simulink model "MSAS Project Part 2.2"  (R2023b)
settings: Solver=ode15s  StartTime=0.0  StopTime=Period  RelTol=1e-9  AbsTol=1e-9
undefined symbols (not defined in the file or in its folder): accelerometer, amplifier, drag, thruster, valve
libraries: fl_lib x15, nesl_utility x10, ee_lib x1
settings Model: Creator=matte  LastModifiedBy=matte

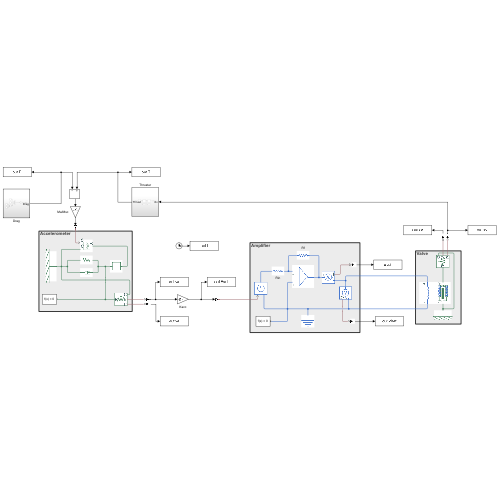
[thumbnail: Simulink's stored preview of the top-level diagram]
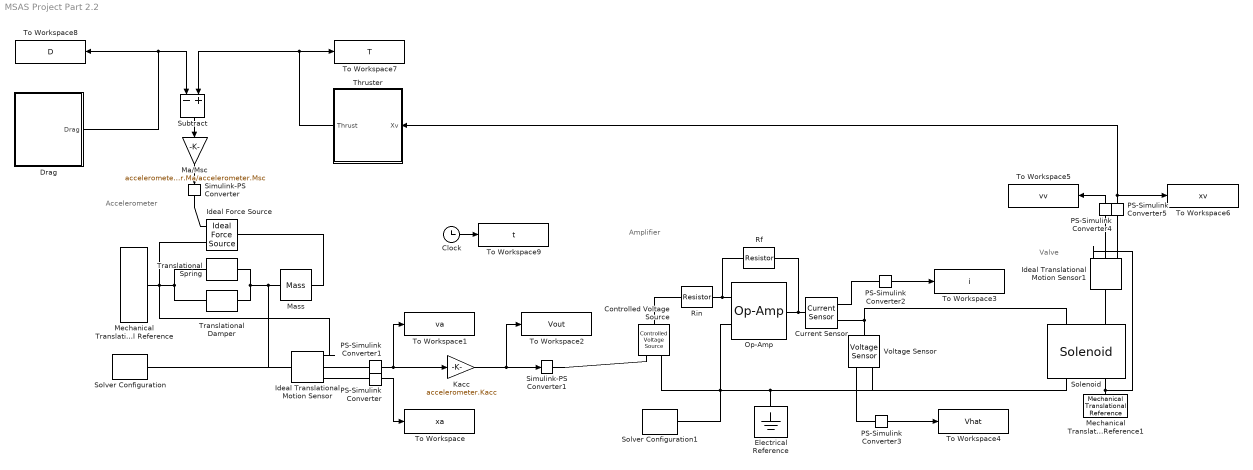
== system MSAS Project Part 2.2 ==
  note: Valve
  note: Amplifier
  note: Accelerometer
  Clock : Clock
  Controlled Voltage Source : fl_lib/Electrical/Electrical Sources/Controlled Voltage Source
  Current Sensor : fl_lib/Electrical/Electrical Sensors/Current Sensor
  Drag : Subsystem
  Electrical Reference : fl_lib/Electrical/Electrical Elements/Electrical Reference
  Ideal Force Source : fl_lib/Mechanical/Mechanical Sources/Ideal Force Source
  Ideal Translational Motion Sensor : fl_lib/Mechanical/Mechanical Sensors/Ideal Translational Motion Sensor  reference=foundation.enum.MeasurementReference.difference  acceleration_port=false  velocity_port=true  position_port=true  offset=0 m
  Ideal Translational Motion Sensor1 : fl_lib/Mechanical/Mechanical Sensors/Ideal Translational Motion Sensor  reference=foundation.enum.MeasurementReference.difference  acceleration_port=false  velocity_port=true  position_port=true  offset=0 m
  Kacc : Gain  Gain=accelerometer.Kacc
  Ma/Msc : Gain  Gain=accelerometer.Ma/accelerometer.Msc
  Mass : fl_lib/Mechanical/Translational Elements/Mass  mass=accelerometer.Ma kg  num_ports=foundation.enum.numPorts2.two  v_specify=off  v_priority=High  v=0 m/s  v_nominal_specify=off  v_nominal_unit=m/s  v_nominal_value=1  f_specify=off  f_priority=None  f=0 N  f_nominal_specify=off  f_nominal_unit=N  f_nominal_value=1
      settings: InternalSimscapePortConfiguration="{\"Bottom\":[],\"Left\":[{\"id\":\"M\",\"label\":\"\",\"type\":\"foundation.mechanical.translational.translational\"}],\"Right\":[{\"id\":\"N\",\"label\":\"\",\"type\":\"foundation.mechanical.translational.translational\"}],\"Top\":[]}"
  Mechanical Translational Reference : fl_lib/Mechanical/Translational Elements/Mechanical Translational Reference
  Mechanical Translational Reference1 : fl_lib/Mechanical/Translational Elements/Mechanical Translational Reference
  Op-Amp : fl_lib/Electrical/Electrical Elements/Op-Amp  outI_specify=off  outI_priority=None  outI=0 A  outI_nominal_specify=off  outI_nominal_unit=A  outI_nominal_value=1
  PS-Simulink Converter{,1..5} (6 alike) : nesl_utility/PS-Simulink Converter  PhysicalDomain=network_engine_domain  SubClassName=ps_output  LeftPortType=input  RightPortType=output  PseudoPeriodic=off  Frequencies=[]  VectorFormat=inherit  Unit=inherit  AffineConversion=off
  Rf : fl_lib/Electrical/Electrical Elements/Resistor  R=amplifier.Rf Ohm  i_specify=off  i_priority=None  i=0 A  i_nominal_specify=off  i_nominal_unit=A  i_nominal_value=1  v_specify=off  v_priority=None  v=0 V  v_nominal_specify=off  v_nominal_unit=V  v_nominal_value=1
  Rin : fl_lib/Electrical/Electrical Elements/Resistor  R=amplifier.Rin Ohm  i_specify=off  i_priority=None  i=0 A  i_nominal_specify=off  i_nominal_unit=A  i_nominal_value=1  v_specify=off  v_priority=None  v=0 V  v_nominal_specify=off  v_nominal_unit=V  v_nominal_value=1
  Simulink-PS Converter : nesl_utility/Simulink-PS Converter  PhysicalDomain=network_engine_domain  SubClassName=ps_input  LeftPortType=input  RightPortType=output  PseudoPeriodic=off  Frequencies=[]  NoiseDistribution=none  NoiseParameters=[]  Unit=1  AffineConversion=off  FilteringAndDerivatives=provide  SimscapeFilterOrder=1  InputFilterTimeConstant=0.001  UdotUserProvided=0
  Simulink-PS Converter1 : nesl_utility/Simulink-PS Converter  PhysicalDomain=network_engine_domain  SubClassName=ps_input  LeftPortType=input  RightPortType=output  PseudoPeriodic=off  Frequencies=[]  NoiseDistribution=none  NoiseParameters=[]  Unit=1  AffineConversion=off  FilteringAndDerivatives=provide  SimscapeFilterOrder=1  InputFilterTimeConstant=0.001  UdotUserProvided=0
  Solenoid : ee_lib/Electromechanical/Mechatronic Actuators/Solenoid  motionDirection=ee.enum.actuators.solenoidDirection.away  F12=[9000, 12] N  X12=[0, 0.1] mm  Vdc=0.6 mV  Imax=0.1 A  K=valve.kv N/m  Xzero=valve.xvMax m  lam=valve.bv N*s/m  Mass=valve.Mv kg  Xmax=0.1 mm  K_endstop=0.12*1e6 N/m  D_endstop=1e4 N*s/m  i_specify=on  i_priority=High  i=0 A  i_nominal_specify=off  i_nominal_unit=A  i_nominal_value=1  x_specify=on  x_priority=High  x=valve.xvMax m  x_nominal_specify=on  x_nominal_unit=m  x_nominal_value=valve.xvMax  vel_specify=off  vel_priority=None  vel=0 mm/s  vel_nominal_specify=off  vel_nominal_unit=mm/s  vel_nominal_value=1  F_specify=off  F_priority=None  F=0 N  F_nominal_specify=off  F_nominal_unit=N  F_nominal_value=1  v_L_specify=off  v_L_priority=None  v_L=0 V  v_L_nominal_specify=off  v_L_nominal_unit=V  v_L_nominal_value=1  magnetic_force_specify=off  magnetic_force_priority=None  magnetic_force=0 N  magnetic_force_nominal_specify=off  magnetic_force_nominal_unit=N  magnetic_force_nominal_value=1  alpha=3.93e-3 1/K  Tmeas=25 degC  thermal_mass=100 J/K  temperature_specify=off  temperature_priority=High  temperature=25 degC  temperature_nominal_specify=off  temperature_nominal_unit=degC  temperature_nominal_value=1  Q_specify=off  Q_priority=None  Q=0 W  Q_nominal_specify=off  Q_nominal_unit=W  Q_nominal_value=1
      settings: InternalSimscapePortConfiguration="{\"Bottom\":[],\"Left\":[{\"id\":\"p\",\"label\":\"+\",\"type\":\"foundation.electrical.electrical\"},{\"id\":\"R\",\"label\":\"R\",\"type\":\"foundation.mechanical.translational.translational\"}],\"Right\":[{\"id\":\"n\",\"label\":\"-\",\"type\":\"foundation.electrical.electrical\"},{\"id\":\"C\",\"label\":\"C\",\"type\":\"foundation.mechanical.translational.translational\"}],\"Top\":[]}"
  Solver Configuration : nesl_utility/Solver Configuration  PhysicalDomain=network_engine_domain  SubClassName=solver  LeftPortType=input  RightPortType=generic  Tones=[]  Harmonics=[]  SimulateNoise=off  Profile=off  UseLocalSampling=off  EnableSwitchedLinearOptims=on  FrequencyDomain=off  UseCCode=off  RelTol=0.001  AbsTol=0.001  MinStep=1e-09  ToWorkspace=off  RevertToSquareIcSolve=off  NumHomotopyIterations=100  PhasorMode=off  PhasorModeNumHarmonics=1  ConsistencySolver=NEWTON_XTOL_AFTER_FTOL  IndexReductionMethod=DerivativeReplacement  DoDC=off  ResidualTolerance=1e-09  ConsistencyTolSource=GLOBAL  ConsistencyAbsTol=0.001  ConsistencyRelTol=0.001  ConsistencyTolFactor=0.001  UseLocalSolver=off  LocalSolverChoice=NE_BACKWARD_EULER_ADVANCER  ResolveIndetEquations=on  FunctionEvalNumThread=1  LocalSolverSampleTime=0.001  DoFixedCost=off  MaxNonlinIter=3  MaxModeIter=2  ComputeImpulses=off  ImpulseIterations=2  LinearAlgebra=auto  LinearAlgebraNumThread=0  EquationFormulation=NE_TIME_EF  DelaysMemoryBudget=1024  AutomaticFiltering=on  FilteringTimeConstant=0.001  PartitionStorageMethod=AS_NEEDED  PartitionMemoryBudget=1024  PartitionMethod=ROBUST  MultibodyUseLocalSolver=off  MultibodyLocalSolverChoice=ODE1  MultibodyLocalSolverSampleTime=0.001
  Solver Configuration1 : nesl_utility/Solver Configuration  PhysicalDomain=network_engine_domain  SubClassName=solver  LeftPortType=input  RightPortType=generic  Tones=[]  Harmonics=[]  SimulateNoise=off  Profile=off  UseLocalSampling=off  EnableSwitchedLinearOptims=on  FrequencyDomain=off  UseCCode=off  RelTol=0.001  AbsTol=0.001  MinStep=1e-09  ToWorkspace=off  RevertToSquareIcSolve=off  NumHomotopyIterations=100  PhasorMode=off  PhasorModeNumHarmonics=1  ConsistencySolver=NEWTON_XTOL_AFTER_FTOL  IndexReductionMethod=DerivativeReplacement  DoDC=off  ResidualTolerance=1e-09  ConsistencyTolSource=GLOBAL  ConsistencyAbsTol=0.001  ConsistencyRelTol=0.001  ConsistencyTolFactor=0.001  UseLocalSolver=off  LocalSolverChoice=NE_BACKWARD_EULER_ADVANCER  ResolveIndetEquations=on  FunctionEvalNumThread=1  LocalSolverSampleTime=0.001  DoFixedCost=off  MaxNonlinIter=3  MaxModeIter=2  ComputeImpulses=off  ImpulseIterations=2  LinearAlgebra=auto  LinearAlgebraNumThread=0  EquationFormulation=NE_TIME_EF  DelaysMemoryBudget=1024  AutomaticFiltering=on  FilteringTimeConstant=0.001  PartitionStorageMethod=AS_NEEDED  PartitionMemoryBudget=1024  PartitionMethod=ROBUST  MultibodyUseLocalSolver=off  MultibodyLocalSolverChoice=ODE1  MultibodyLocalSolverSampleTime=0.001
  Subtract : Sum  Inputs=-+
  Thruster : Subsystem
  To Workspace : ToWorkspace  VariableName=xa  SampleTime=-1
  To Workspace1 : ToWorkspace  VariableName=va  SampleTime=-1
      settings: Save2DSignal=2-D array (concatenate along first dimension)
  To Workspace2 : ToWorkspace  VariableName=Vout  SampleTime=-1
      settings: Save2DSignal=2-D array (concatenate along first dimension)
  To Workspace3 : ToWorkspace  VariableName=i  SampleTime=-1
  To Workspace4 : ToWorkspace  VariableName=Vhat  SampleTime=-1
  To Workspace5 : ToWorkspace  VariableName=vv  SampleTime=-1
  To Workspace6 : ToWorkspace  VariableName=xv  SampleTime=-1
  To Workspace7 : ToWorkspace  VariableName=T  SampleTime=-1
  To Workspace8 : ToWorkspace  VariableName=D  SampleTime=-1
  To Workspace9 : ToWorkspace  VariableName=t  SampleTime=-1
  Translational Damper : fl_lib/Mechanical/Translational Elements/Translational Damper  D=accelerometer.ba N*s/m  v_specify=off  v_priority=None  v=0 m/s  v_nominal_specify=off  v_nominal_unit=m/s  v_nominal_value=1  f_specify=off  f_priority=None  f=0 N  f_nominal_specify=off  f_nominal_unit=N  f_nominal_value=1
  Translational Spring : fl_lib/Mechanical/Translational Elements/Translational Spring  spr_rate=accelerometer.ka N/m  v_specify=off  v_priority=None  v=0 m/s  v_nominal_specify=off  v_nominal_unit=m/s  v_nominal_value=1  f_specify=off  f_priority=None  f=0 N  f_nominal_specify=off  f_nominal_unit=N  f_nominal_value=1  x_specify=off  x_priority=High  x=0 m  x_nominal_specify=off  x_nominal_unit=m  x_nominal_value=1
  Voltage Sensor : fl_lib/Electrical/Electrical Sensors/Voltage Sensor
  wires:
  PS-Simulink Converter/1 -> To Workspace/1
  PS-Simulink Converter3/1 -> To Workspace4/1
  PS-Simulink Converter4/1 -> To Workspace5/1
  Subtract/1 -> Ma/Msc/1
  Thruster/1(Thrust) -> Subtract/2, To Workspace7/1
  Drag/1(Drag) -> Subtract/1, To Workspace8/1
  PS-Simulink Converter1/1 -> Kacc/1, To Workspace1/1
  PS-Simulink Converter5/1 -> Thruster/1(Xv), To Workspace6/1
  PS-Simulink Converter2/1 -> To Workspace3/1
  Ma/Msc/1 -> Simulink-PS Converter/1
  Kacc/1 -> Simulink-PS Converter1/1, To Workspace2/1
  Clock/1 -> To Workspace9/1
  connections:
  Simulink-PS Converter/RConn1 -- Ideal Force Source/RConn1
  Mechanical Translational Reference/LConn1 -- Translational Damper/RConn1 -- Translational Spring/RConn1 -- Ideal Force Source/RConn2 -- Ideal Translational Motion Sensor/RConn1
  Ideal Force Source/LConn1 -- Mass/LConn1
  Translational Damper/LConn1 -- Translational Spring/LConn1 -- Solver Configuration/RConn1 -- Ideal Translational Motion Sensor/LConn1 -- Mass/RConn1
  PS-Simulink Converter/LConn1 -- Ideal Translational Motion Sensor/RConn3
  Simulink-PS Converter1/RConn1 -- Controlled Voltage Source/RConn1
  Controlled Voltage Source/LConn1 -- Rin/LConn1
  Op-Amp/LConn2 -- Rf/RConn1 -- Rin/RConn1
  Rf/LConn1 -- Current Sensor/LConn1 -- Op-Amp/RConn1
  Controlled Voltage Source/RConn2 -- Solver Configuration1/RConn1 -- Solenoid/RConn1 -- Voltage Sensor/RConn2 -- Electrical Reference/LConn1 -- Op-Amp/LConn1
  PS-Simulink Converter2/LConn1 -- Current Sensor/RConn1
  Current Sensor/RConn2 -- Solenoid/LConn1 -- Voltage Sensor/LConn1
  Voltage Sensor/RConn1 -- PS-Simulink Converter3/LConn1
  Mechanical Translational Reference1/LConn1 -- Ideal Translational Motion Sensor1/RConn1 -- Solenoid/RConn2
  Ideal Translational Motion Sensor1/LConn1 -- Solenoid/LConn2
  PS-Simulink Converter1/LConn1 -- Ideal Translational Motion Sensor/RConn2
  Ideal Translational Motion Sensor1/RConn3 -- PS-Simulink Converter5/LConn1
  Ideal Translational Motion Sensor1/RConn2 -- PS-Simulink Converter4/LConn1

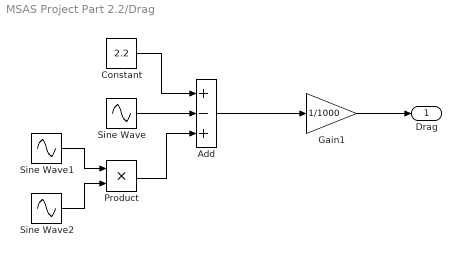
== system MSAS Project Part 2.2/Drag ==
  Add : Sum  Inputs=+-+
  Constant : Constant  Value=2.2
  Gain1 : Gain  Gain=1/1000
  Product : Product
  Sine Wave : Sin  Frequency=drag.omegaS  Phase=pi/2  SampleTime=0
  Sine Wave1 : Sin  Amplitude=1.2  Frequency=drag.omegaO  SampleTime=0
  Sine Wave2 : Sin  Frequency=drag.omegaO  Phase=pi/2  SampleTime=0
  Drag : Outport
  wires:
  Add/1 -> Gain1/1
  Constant/1 -> Add/1
  Gain1/1 -> Drag/1
  Sine Wave/1 -> Add/2
  Sine Wave1/1 -> Product/1
  Sine Wave2/1 -> Product/2
  Product/1 -> Add/3

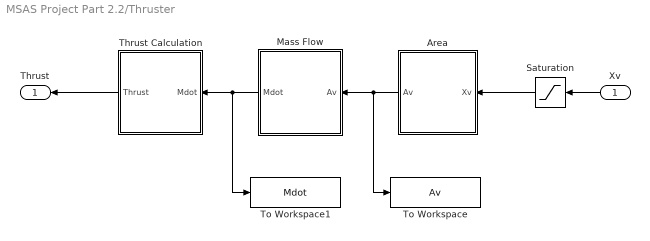
== system MSAS Project Part 2.2/Thruster ==
  Xv : Inport
  Area : Subsystem
  Mass Flow : Subsystem
  Saturation : Saturate  UpperLimit=valve.xvMax  LowerLimit=0
  Thrust Calculation : Subsystem
  To Workspace : ToWorkspace  VariableName=Av  SampleTime=-1
  To Workspace1 : ToWorkspace  VariableName=Mdot  SampleTime=-1
  Thrust : Outport
  wires:
  Area/1(Av) -> To Workspace/1, Mass Flow/1(Av)
  Mass Flow/1(Mdot) -> To Workspace1/1, Thrust Calculation/1(Mdot)
  Xv/1 -> Saturation/1
  Thrust Calculation/1(Thrust) -> Thrust/1
  Saturation/1 -> Area/1(Xv)

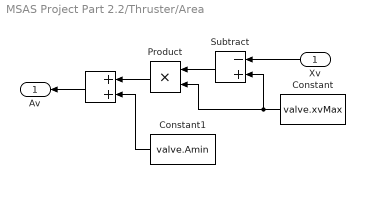
== system MSAS Project Part 2.2/Thruster/Area ==
  Xv : Inport
  " " : Sum
  Constant : Constant  Value=valve.xvMax
  Constant1 : Constant  Value=valve.Amin
  Product : Product
  Subtract : Sum  Inputs=-+
  Av : Outport
  wires:
  Product/1 -> " "/1
  Constant1/1 -> " "/2
  Constant/1 -> Subtract/2, Product/2
  Subtract/1 -> Product/1
  " "/1 -> Av/1
  Xv/1 -> Subtract/1

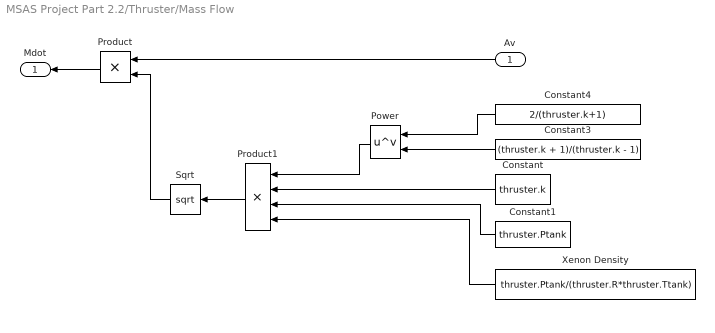
== system MSAS Project Part 2.2/Thruster/Mass Flow ==
  Av : Inport
  Constant : Constant  Value=thruster.k
  Constant1 : Constant  Value=thruster.Ptank
  Constant3 : Constant  Value=(thruster.k + 1)/(thruster.k - 1)
  Constant4 : Constant  Value=2/(thruster.k+1)
  Power : Math  Operator=pow
  Product : Product
  Product1 : Product  Inputs=4
  Sqrt : Sqrt
  Xenon Density : Constant  Value=thruster.Ptank/(thruster.R*thruster.Ttank)
  Mdot : Outport
  wires:
  Product/1 -> Mdot/1
  Av/1 -> Product/1
  Sqrt/1 -> Product/2
  Product1/1 -> Sqrt/1
  Xenon Density/1 -> Product1/4
  Constant1/1 -> Product1/3
  Constant/1 -> Product1/2
  Constant3/1 -> Power/2
  Constant4/1 -> Power/1
  Power/1 -> Product1/1

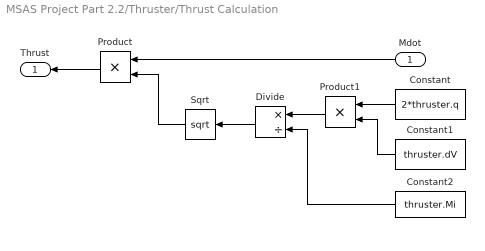
== system MSAS Project Part 2.2/Thruster/Thrust Calculation ==
  Mdot : Inport
  Constant : Constant  Value=2*thruster.q
  Constant1 : Constant  Value=thruster.dV
  Constant2 : Constant  Value=thruster.Mi
  Divide : Product  Inputs=*/
  Product : Product
  Product1 : Product
  Sqrt : Sqrt
  Thrust : Outport
  wires:
  Mdot/1 -> Product/1
  Product/1 -> Thrust/1
  Constant1/1 -> Product1/2
  Constant/1 -> Product1/1
  Product1/1 -> Divide/1
  Constant2/1 -> Divide/2
  Divide/1 -> Sqrt/1
  Sqrt/1 -> Product/2
